simulink subsystem "AxleCompliances"  (R2023b)
settings: Solver=VariableStepAuto  StartTime=0.0  StopTime=10.0  RelTol=1e-3
undefined symbols (not defined in the file): PlntDriveshftDamp, PlntDriveshftStiff
libraries: autolibsharedcoupling x2
settings Model: Creator=The MathWorks, Inc.  LastModifiedBy=The MathWorks, Inc.
settings DebuggingCC: SubsystemReferenceDiagnosticForUnitTest=warning

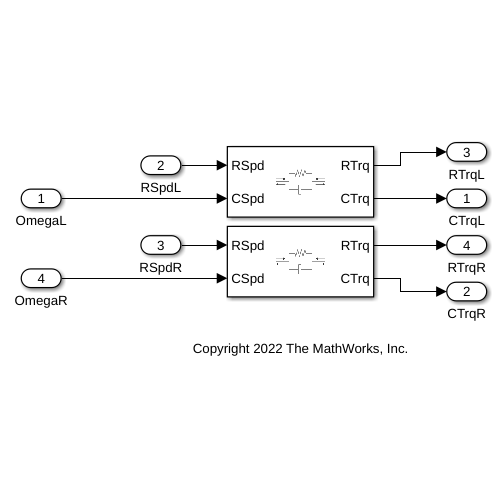
[thumbnail: Simulink's stored preview of the top-level diagram]
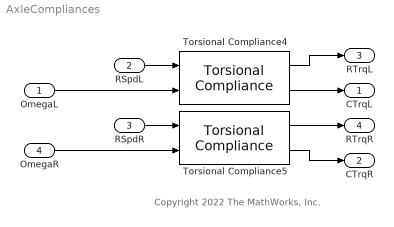
== system AxleCompliances ==
  note: Copyright 2022 The MathWorks, Inc.
  OmegaL : Inport
  RSpdL : Inport  Port=2
  RSpdR : Inport  Port=3
  OmegaR : Inport  Port=4
  Torsional Compliance4 : autolibsharedcoupling/Torsional Compliance  port_config=Simulink  extInfo=off  k=PlntDriveshftStiff  b=PlntDriveshftDamp  theta_o=PlntDriveshftInitDeflect  domega_o=PlntDriveshftInitVel  omega_c=PlntDriveshftDampCutoffFreq  blkID=0  aMode=6
  Torsional Compliance5 : autolibsharedcoupling/Torsional Compliance  port_config=Simulink  extInfo=off  k=PlntDriveshftStiff  b=PlntDriveshftDamp  theta_o=PlntDriveshftInitDeflect  domega_o=PlntDriveshftInitVel  omega_c=PlntDriveshftDampCutoffFreq  blkID=0  aMode=6
  CTrqL : Outport
  CTrqR : Outport  Port=2
  RTrqL : Outport  Port=3
  RTrqR : Outport  Port=4
  wires:
  OmegaR/1 -> Torsional Compliance5/2
  Torsional Compliance4/1 -> RTrqL/1
  Torsional Compliance5/1 -> RTrqR/1
  Torsional Compliance5/2 -> CTrqR/1
  OmegaL/1 -> Torsional Compliance4/2
  Torsional Compliance4/2 -> CTrqL/1
  RSpdR/1 -> Torsional Compliance5/1
  RSpdL/1 -> Torsional Compliance4/1
